simulink model "Test_FourMotor_PID_Ave"  (R2025a)
settings: Solver=ode4  StartTime=0.0  StopTime=2  FixedStep=60e-6  RelTol=1e-3
values from neighbouring files (symbols this model uses):
  Ts = 2e-6    (= 2e-06)    [param.m]
  ts_vec = 60e-6    (= 6e-05)    [param.m]
undefined symbols (not defined in the file or in its folder): DiscIntNeverNeededParam, gcbh, HEV_Param, Limit, magnitude, motorctrl, RPM, sps_rtmsupport
libraries: fl_lib x39, spsCurrentMeasurementLib x26, spsIdealSwitchLib x24, nesl_utility x22, spsVoltageMeasurementLib x21, simulink_extras x13, spsControlledCurrentSourceLib x12, spsControlledVoltageSourceLib x9, slpidlib x7, simulink x6, Uav_Electrical_lib x5, spsSeriesRLCBranchLib x4
(part 3 of 5)

== system Test_FourMotor_PID_Ave/Detailed/Synchronous Motor & Drive1/Torque limitation ==
  N rad/s : Inport
  Torque : Inport  Port=2
  Abs1 : Abs
  Gain : Gain  Gain=-1
  Saturation Dynamic : simulink/Discontinuities/Saturation Dynamic  OutMin=[]  OutMax=[]  OutDataTypeStr=Inherit: Same as second input  OutDataType=sfix(16)  OutScaling=2^-10  DoSatur=off
  Torque vs speed profile : Lookup  InputValues=HEV_Param.Motor.TorqSpdLUT.SpeedRPM*pi/30  Table=HEV_Param.Motor.TorqSpdLUT.TorqueNm  LookUpMeth=Interpolation-Use End Values  SaturateOnIntegerOverflow=off
  torque : Outport  VectorParamsAs1DForOutWhenUnconnected=off
  wires:
  Gain/1 -> Saturation Dynamic/3
  Torque/1 -> Saturation Dynamic/2
  Saturation Dynamic/1 -> torque/1
  Torque vs speed profile/1 -> Gain/1, Saturation Dynamic/1
  Abs1/1 -> Torque vs speed profile/1
  N rad/s/1 -> Abs1/1

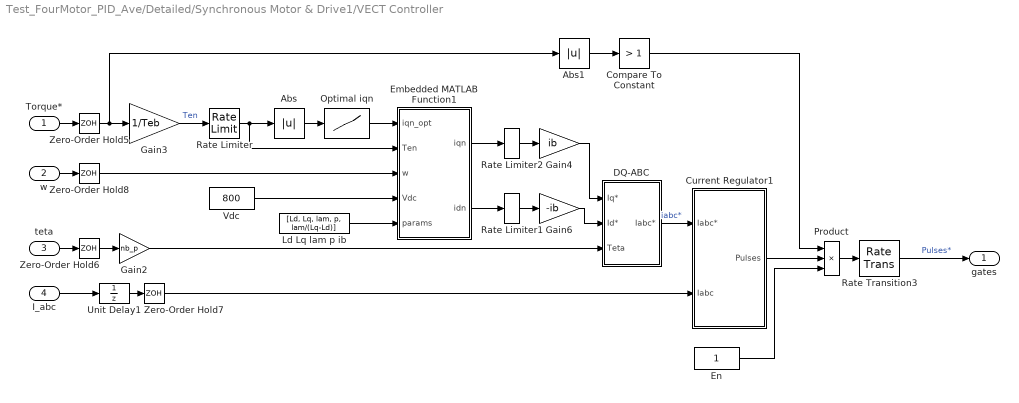
== system Test_FourMotor_PID_Ave/Detailed/Synchronous Motor & Drive1/VECT Controller ==
  Torque* : Inport
  w : Inport  Port=2
  teta : Inport  Port=3
  I_abc : Inport  Port=4
  Abs : Abs  SaturateOnIntegerOverflow=off
  Abs1 : Abs  SaturateOnIntegerOverflow=off
  Compare To Constant : simulink/Logic and Bit Operations/Compare To Constant  relop=>  const=1  OutDataTypeStr=uint8
  Current Regulator1 : Subsystem
  DQ-ABC : Subsystem
  Embedded MATLAB Function1 : MATLAB Function  TreatAsAtomicUnit=on  SystemSampleTime=Ts_vect
  En : Constant
  Gain2 : Gain  Gain=nb_p  SaturateOnIntegerOverflow=on  OutDataTypeStr=Inherit: Same as input  ParamDataTypeStr=Inherit: Same as input
  Gain3 : Gain  Gain=1/Teb  SaturateOnIntegerOverflow=on  OutDataTypeStr=Inherit: Same as input  ParamDataTypeStr=Inherit: Same as input
  Gain4 : Gain  Gain=ib  SaturateOnIntegerOverflow=on  OutDataTypeStr=Inherit: Same as input  ParamDataTypeStr=Inherit: Same as input
  Gain6 : Gain  Gain=-ib  SaturateOnIntegerOverflow=on  OutDataTypeStr=Inherit: Same as input  ParamDataTypeStr=Inherit: Same as input
  Ld Lq lam p ib : Constant  Value=[Ld, Lq, lam, p, lam/(Lq-Ld)]
  Optimal iqn : Lookup  InputValues=ten  Table=iqn  SaturateOnIntegerOverflow=off
  Product : Product  Inputs=3  RndMeth=Zero
  Rate Limiter : RateLimiter  RisingSlewLimit=10  FallingSlewLimit=-10  LinearizeAsGain=off
  Rate Limiter1 : RateLimiter  RisingSlewLimit=100  FallingSlewLimit=-100  SampleTimeMode=inherited
  Rate Limiter2 : RateLimiter  RisingSlewLimit=100  FallingSlewLimit=-100  SampleTimeMode=inherited
  Rate Transition3 : RateTransition
  Unit Delay1 : UnitDelay  SampleTime=-1  HasFrameUpgradeWarning=on
  Vdc : Constant  Value=800
  Zero-Order Hold{5..8} (4 alike) : ZeroOrderHold  SampleTime=Ts_vect
  gates : Outport  VectorParamsAs1DForOutWhenUnconnected=off
  wires:
  Abs1/1 -> Compare To Constant/1
  Compare To Constant/1 -> Product/1
  En/1 -> Product/3
  Current Regulator1/1(Pulses) -> Product/2
  Unit Delay1/1 -> Zero-Order Hold7/1
  Zero-Order Hold7/1 -> Current Regulator1/2(Iabc)
  teta/1 -> Zero-Order Hold6/1
  Zero-Order Hold6/1 -> Gain2/1
  Gain2/1 -> DQ-ABC/3(Teta)
  DQ-ABC/1(Iabc*) -> Current Regulator1/1(Iabc*)  "iabc*"
  I_abc/1 -> Unit Delay1/1
  Torque*/1 -> Zero-Order Hold5/1
  Gain4/1 -> DQ-ABC/1("Iq* ")
  Gain6/1 -> DQ-ABC/2("Id* ")
  Zero-Order Hold5/1 -> Abs1/1, Gain3/1
  w/1 -> Zero-Order Hold8/1
  Embedded MATLAB Function1/2(idn) -> Rate Limiter1/1
  Gain3/1 -> Rate Limiter/1  "Ten"
  Zero-Order Hold8/1 -> Embedded MATLAB Function1/3(w)
  Ld Lq lam p ib/1 -> Embedded MATLAB Function1/5(params)
  Embedded MATLAB Function1/1(iqn) -> Rate Limiter2/1
  Optimal iqn/1 -> Embedded MATLAB Function1/1(iqn_opt)
  Abs/1 -> Optimal iqn/1
  Vdc/1 -> Embedded MATLAB Function1/4(Vdc)
  Rate Transition3/1 -> gates/1  "Pulses*"
  Product/1 -> Rate Transition3/1
  Rate Limiter2/1 -> Gain4/1
  Rate Limiter1/1 -> Gain6/1
  Rate Limiter/1 -> Abs/1, Embedded MATLAB Function1/2(Ten)

== system Test_FourMotor_PID_Ave/Detailed/Synchronous Motor & Drive2/GF ==
  In1 : Inport
  Out1 : Outport  VectorParamsAs1DForOutWhenUnconnected=off
  tag scope: Mot_TReq_SYS_2=global
  wires:
  In1/1 -> Out1/1, [Mot_TReq_SYS_2]

== system Test_FourMotor_PID_Ave/Detailed/Synchronous Motor & Drive2/Measures ==
  Current Measurement : spsCurrentMeasurementLib/Current Measurement  Tag=PoWeRsYsTeMmEaSuReMeNt  PhasorSimulation=off  OutputType=Magnitude  PSBequivalent=0
      settings: AttributesFormatString=\n
  Current Measurement1 : spsCurrentMeasurementLib/Current Measurement  Tag=PoWeRsYsTeMmEaSuReMeNt  PhasorSimulation=off  OutputType=Magnitude  PSBequivalent=0
      settings: AttributesFormatString=\n
  Current Measurement2 : spsCurrentMeasurementLib/Current Measurement  Tag=PoWeRsYsTeMmEaSuReMeNt  PhasorSimulation=off  OutputType=Magnitude  PSBequivalent=0
      settings: AttributesFormatString=\n
  Mux1 : Mux  Inputs=3
  Ta : PMIOPort  Side=Left
  Tb : PMIOPort  Port=2  Side=Left
  Tc : PMIOPort  Port=3  Side=Left
  Mta : PMIOPort  Port=4  Side=Right
  Mtb : PMIOPort  Port=5  Side=Right
  Mtc : PMIOPort  Port=6  Side=Right
  I_abc : Outport  VectorParamsAs1DForOutWhenUnconnected=off
  wires:
  Current Measurement1/1 -> Mux1/2
  Current Measurement/1 -> Mux1/1
  Current Measurement2/1 -> Mux1/3
  Mux1/1 -> I_abc/1
  connections:
  Current Measurement1/RConn1 -- Mtb/RConn1
  Tb/RConn1 -- Current Measurement1/LConn1
  Current Measurement/RConn1 -- Mta/RConn1
  Ta/RConn1 -- Current Measurement/LConn1
  Tc/RConn1 -- Current Measurement2/LConn1
  Current Measurement2/RConn1 -- Mtc/RConn1

== system Test_FourMotor_PID_Ave/Detailed/Synchronous Motor & Drive2/Subsystem ==
  In : Inport
  "+ -> -1" : Gain  Gain=30/pi
  Bus Selector : BusSelector  OutputSignals=Stator current is_a (A),Rotor speed wm (rad/s),Electromagnetic torque Te (N*m)
  Mux1 : Mux  Inputs=2
  Mux2 : Mux  Inputs=3
  Out : Outport  VectorParamsAs1DForOutWhenUnconnected=off
  tag scope: MotorDrive_2=global
  wires:
  In/1 -> Bus Selector/1, Out/1
  "+ -> -1"/1 -> Mux2/2
  [Mot_TReq_SYS_2] -> Mux1/2
  Bus Selector/2 -> "+ -> -1"/1  "<Rotor speed wm (rad/s)>"
  Bus Selector/3 -> Mux1/1  "<Electromagnetic torque Te (N*m)>"
  Mux1/1 -> Mux2/3
  Bus Selector/1 -> Mux2/1  "<Stator current is_a (A)>"
  Mux2/1 -> [MotorDrive_2]

== system Test_FourMotor_PID_Ave/Detailed/Synchronous Motor & Drive2/Subsystem1 ==
  Sig : Inport
  Bus Selector : BusSelector  OutputSignals=Electromagnetic torque Te (N*m)
  Ideal Rotational Motion Sensor : fl_lib/Mechanical/Mechanical Sensors/Ideal Rotational Motion Sensor  reference=foundation.enum.MeasurementReference.difference  acceleration_port=false  velocity_port=true  position_port=true  wrap_angle=simscape.enum.onoff.off  offset=0 rad
  Ideal Torque Source : fl_lib/Mechanical/Mechanical Sources/Ideal Torque Source
  Mechanical Rotational Reference : fl_lib/Mechanical/Rotational Elements/Mechanical Rotational Reference
  Mechanical Rotational Reference1 : fl_lib/Mechanical/Rotational Elements/Mechanical Rotational Reference
  PS-Simulink Converter : nesl_utility/PS-Simulink Converter  PhysicalDomain=network_engine_domain  SubClassName=ps_output  LeftPortType=input  RightPortType=output  PseudoPeriodic=off  Frequencies=[]  VectorFormat=1-D array  Unit=rad/s  AffineConversion=off
  Scope : Scope
      settings: ActiveDisplayYMinimum=-14.945816065975556  ActiveDisplayYMaximum=38.271093163037733  DataLoggingVariableName=ScopeData6
  Simulink-PS Converter : nesl_utility/Simulink-PS Converter  PhysicalDomain=network_engine_domain  SubClassName=ps_input  LeftPortType=input  RightPortType=output  PseudoPeriodic=off  Frequencies=[]  NoiseDistribution=none  NoiseParameters=[]  Unit=1  AffineConversion=off  FilteringAndDerivatives=zero  SimscapeFilterOrder=1  InputFilterTimeConstant=0.005  UdotUserProvided=0
  Sh : PMIOPort  Side=Right
  Spd : Outport  VectorParamsAs1DForOutWhenUnconnected=off
  wires:
  PS-Simulink Converter/1 -> Spd/1
  Sig/1 -> Bus Selector/1
  Bus Selector/1 -> Scope/1, Simulink-PS Converter/1  "<Electromagnetic torque Te (N*m)>"
  connections:
  Simulink-PS Converter/RConn1 -- Ideal Torque Source/RConn1
  PS-Simulink Converter/LConn1 -- Ideal Rotational Motion Sensor/RConn2
  Ideal Rotational Motion Sensor/LConn1 -- Sh/RConn1 -- Ideal Torque Source/LConn1
  Mechanical Rotational Reference1/LConn1 -- Ideal Torque Source/RConn2
  Mechanical Rotational Reference/LConn1 -- Ideal Rotational Motion Sensor/RConn1

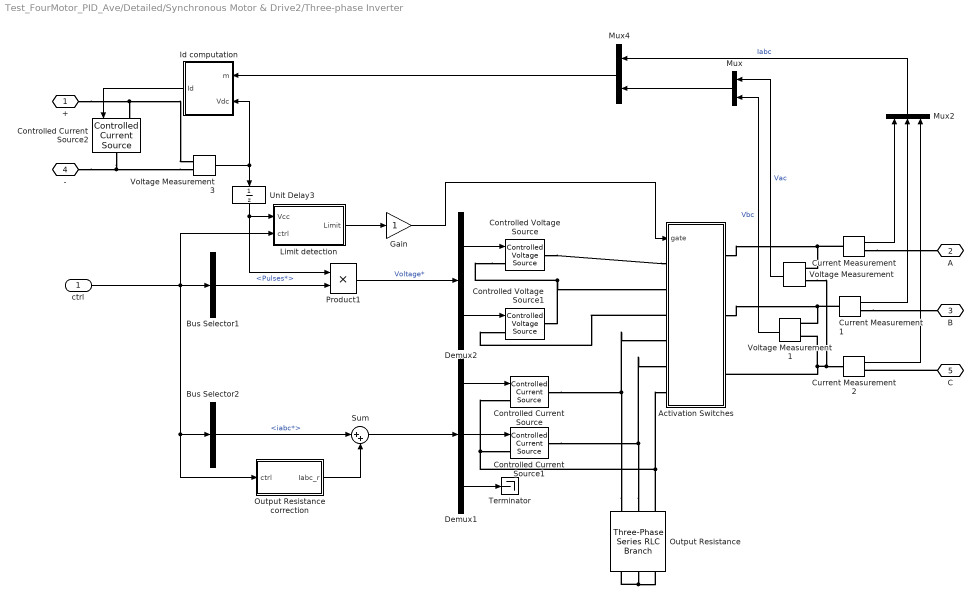
== system Test_FourMotor_PID_Ave/Detailed/Synchronous Motor & Drive2/Three-phase Inverter ==
  ctrl : Inport
  Activation Switches : Subsystem
  Bus Selector1 : BusSelector  OutputSignals=Signals*.Pulses*
  Bus Selector2 : BusSelector  OutputSignals=Signals*.iabc*
  Controlled Current Source : spsControlledCurrentSourceLib/Controlled Current Source  Initialize=on  Source_Type=AC  Amplitude=0  Phase=0  Frequency=0  Measurements=None
  Controlled Current Source1 : spsControlledCurrentSourceLib/Controlled Current Source  Initialize=on  Source_Type=AC  Amplitude=0  Phase=0  Frequency=0  Measurements=None
  Controlled Current Source2 : spsControlledCurrentSourceLib/Controlled Current Source  Initialize=on  Source_Type=AC  Amplitude=0  Phase=0  Frequency=0  Measurements=None
  Controlled Voltage Source : spsControlledVoltageSourceLib/Controlled Voltage Source  Initialize=on  Source_Type=AC  Amplitude=0  Phase=0  Frequency=0  Measurements=None
  Controlled Voltage Source1 : spsControlledVoltageSourceLib/Controlled Voltage Source  Initialize=on  Source_Type=AC  Amplitude=0  Phase=0  Frequency=0  Measurements=None
  Current Measurement : spsCurrentMeasurementLib/Current Measurement  PhasorSimulation=off  OutputType=Complex  PSBequivalent=0
  Current Measurement1 : spsCurrentMeasurementLib/Current Measurement  PhasorSimulation=off  OutputType=Complex  PSBequivalent=0
  Current Measurement2 : spsCurrentMeasurementLib/Current Measurement  PhasorSimulation=off  OutputType=Complex  PSBequivalent=0
  Demux1 : Demux  Outputs=3
      settings: DisplayOption=none
  Demux2 : Demux  Outputs=2
      settings: DisplayOption=none
  Gain : Gain
  Id computation : Subsystem
  Limit detection : Subsystem
  Mux : Mux  Inputs=2
  Mux2 : Mux  Inputs=3
  Mux4 : Mux  Inputs=2
  Output Resistance : spsThreePhaseSeriesRLCBranchLib/Three-Phase Series RLC Branch  LConnTagsString=A|B|C  RConnTagsString=A|B|C  BranchType=R  Resistance=100*Resistance  Inductance=1e-3  Capacitance=1e-6  Measurements=Branch voltages and currents
  Output Resistance correction : Subsystem
  Product1 : Product  RndMeth=Zero
  Sum : Sum  Inputs=|++
  Terminator : Terminator
  Unit Delay3 : UnitDelay  SampleTime=Ts  HasFrameUpgradeWarning=on
  Voltage Measurement : spsVoltageMeasurementLib/Voltage Measurement  PhasorSimulation=off  OutputType=Complex  PSBequivalent=0
  Voltage Measurement1 : spsVoltageMeasurementLib/Voltage Measurement  PhasorSimulation=off  OutputType=Complex  PSBequivalent=0
  Voltage Measurement3 : spsVoltageMeasurementLib/Voltage Measurement  PhasorSimulation=off  OutputType=Complex  PSBequivalent=0
  + : PMIOPort  Side=Right
  A : PMIOPort  Port=2  Side=Left
  B : PMIOPort  Port=3  Side=Left
  - : PMIOPort  Port=4  Side=Right
  C : PMIOPort  Port=5  Side=Left
  wires:
  Current Measurement/1 -> Mux2/1
  Current Measurement1/1 -> Mux2/2
  Voltage Measurement/1 -> Mux/1  "Vac"
  Voltage Measurement1/1 -> Mux/2  "Vbc"
  Mux/1 -> Mux4/2
  Current Measurement2/1 -> Mux2/3
  Mux4/1 -> Id computation/1(m)
  Mux2/1 -> Mux4/1  "Iabc"
  Voltage Measurement3/1 -> Unit Delay3/1, Id computation/2(Vdc)
  Bus Selector1/1 -> Product1/2  "<Pulses*>"
  Demux1/1 -> Controlled Current Source/1
  Demux1/2 -> Controlled Current Source1/1
  Demux1/3 -> Terminator/1
  Demux2/2 -> Controlled Voltage Source1/1
  Demux2/1 -> Controlled Voltage Source/1
  Bus Selector2/1 -> Sum/1  "<iabc*>"
  Limit detection/1(Limit) -> Gain/1
  Sum/1 -> Demux1/1
  Unit Delay3/1 -> Product1/1, Limit detection/1(Vcc)
  ctrl/1 -> Bus Selector1/1, Limit detection/2(ctrl), Bus Selector2/1, Output Resistance correction/1(ctrl)
  Product1/1 -> Demux2/1  "Voltage*"
  Gain/1 -> Activation Switches/1(gate)
  Id computation/1(Id) -> Controlled Current Source2/1
  Output Resistance correction/1("Iabc_r ") -> Sum/2
  connections:
  Voltage Measurement3/LConn1 -- Controlled Current Source2/LConn1 -- +/RConn1
  Voltage Measurement3/LConn2 -- Controlled Current Source2/RConn1 -- -/RConn1
  Activation Switches/LConn6 -- Controlled Current Source/LConn1 -- Controlled Current Source1/LConn1 -- Output Resistance/LConn3
  Output Resistance/RConn1 -- Output Resistance/RConn3 -- Output Resistance/RConn2
  Voltage Measurement/LConn1 -- Activation Switches/RConn1 -- Current Measurement/LConn1
  Output Resistance/LConn1 -- Activation Switches/LConn4 -- Controlled Current Source/RConn1
  Output Resistance/LConn2 -- Activation Switches/LConn5 -- Controlled Current Source1/RConn1
  Voltage Measurement/LConn2 -- Activation Switches/RConn3 -- Voltage Measurement1/LConn2 -- Current Measurement2/LConn1
  Controlled Voltage Source/LConn1 -- Activation Switches/LConn2 -- Controlled Voltage Source1/RConn1
  Voltage Measurement1/LConn1 -- Activation Switches/RConn2 -- Current Measurement1/LConn1
  Current Measurement/RConn1 -- A/RConn1
  Current Measurement1/RConn1 -- B/RConn1
  C/RConn1 -- Current Measurement2/RConn1
  Controlled Voltage Source/RConn1 -- Activation Switches/LConn1
  Activation Switches/LConn3 -- Controlled Voltage Source1/LConn1

== system Test_FourMotor_PID_Ave/Detailed/Synchronous Motor & Drive2/Torque limitation ==
  N rad/s : Inport
  Torque : Inport  Port=2
  Abs1 : Abs
  Gain : Gain  Gain=-1
  Saturation Dynamic : simulink/Discontinuities/Saturation Dynamic  OutMin=[]  OutMax=[]  OutDataTypeStr=Inherit: Same as second input  OutDataType=sfix(16)  OutScaling=2^-10  DoSatur=off
  Torque vs speed profile : Lookup  InputValues=HEV_Param.Motor.TorqSpdLUT.SpeedRPM*pi/30  Table=HEV_Param.Motor.TorqSpdLUT.TorqueNm  LookUpMeth=Interpolation-Use End Values  SaturateOnIntegerOverflow=off
  torque : Outport  VectorParamsAs1DForOutWhenUnconnected=off
  wires:
  Gain/1 -> Saturation Dynamic/3
  Torque/1 -> Saturation Dynamic/2
  Saturation Dynamic/1 -> torque/1
  Torque vs speed profile/1 -> Gain/1, Saturation Dynamic/1
  Abs1/1 -> Torque vs speed profile/1
  N rad/s/1 -> Abs1/1

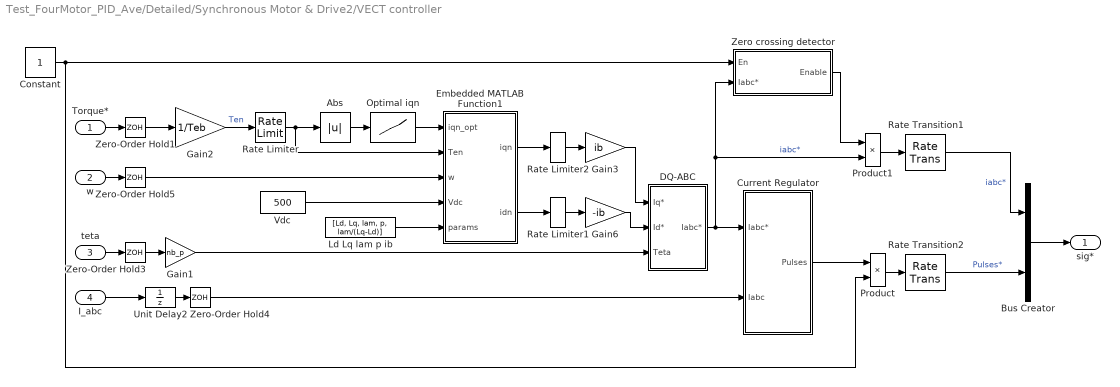
== system Test_FourMotor_PID_Ave/Detailed/Synchronous Motor & Drive2/VECT controller ==
  Torque* : Inport
  w : Inport  Port=2
  teta : Inport  Port=3
  I_abc : Inport  Port=4
  Abs : Abs  SaturateOnIntegerOverflow=off
  Bus Creator : BusCreator  Inputs=2
  Constant : Constant
  Current Regulator : Subsystem
  DQ-ABC : Subsystem
  Embedded MATLAB Function1 : MATLAB Function  TreatAsAtomicUnit=on  SystemSampleTime=Ts_vect
  Gain1 : Gain  Gain=nb_p  SaturateOnIntegerOverflow=on  OutDataTypeStr=Inherit: Same as input  ParamDataTypeStr=Inherit: Same as input
  Gain2 : Gain  Gain=1/Teb  SaturateOnIntegerOverflow=on  OutDataTypeStr=Inherit: Same as input  ParamDataTypeStr=Inherit: Same as input
  Gain3 : Gain  Gain=ib  SaturateOnIntegerOverflow=on  OutDataTypeStr=Inherit: Same as input  ParamDataTypeStr=Inherit: Same as input
  Gain6 : Gain  Gain=-ib  SaturateOnIntegerOverflow=on  OutDataTypeStr=Inherit: Same as input  ParamDataTypeStr=Inherit: Same as input
  Ld Lq lam p ib : Constant  Value=[Ld, Lq, lam, p, lam/(Lq-Ld)]
  Optimal iqn : Lookup  InputValues=ten  Table=iqn  SaturateOnIntegerOverflow=off
  Product : Product  RndMeth=Zero
  Product1 : Product  RndMeth=Zero
  Rate Limiter : RateLimiter  RisingSlewLimit=10  FallingSlewLimit=-10  LinearizeAsGain=off
  Rate Limiter1 : RateLimiter  RisingSlewLimit=100  FallingSlewLimit=-100  SampleTimeMode=inherited
  Rate Limiter2 : RateLimiter  RisingSlewLimit=100  FallingSlewLimit=-100  SampleTimeMode=inherited
  Rate Transition1 : RateTransition
  Rate Transition2 : RateTransition
  Unit Delay2 : UnitDelay  SampleTime=-1  HasFrameUpgradeWarning=on
  Vdc : Constant  Value=500
  Zero crossing detector : Subsystem
  Zero-Order Hold{1,3..5} (4 alike) : ZeroOrderHold  SampleTime=Ts_vect
  sig* : Outport  VectorParamsAs1DForOutWhenUnconnected=off
  wires:
  Unit Delay2/1 -> Zero-Order Hold4/1
  Zero-Order Hold4/1 -> Current Regulator/2(Iabc)
  teta/1 -> Zero-Order Hold3/1
  Zero-Order Hold3/1 -> Gain1/1
  Gain1/1 -> DQ-ABC/3(Teta)
  DQ-ABC/1(Iabc*) -> Current Regulator/1(Iabc*), Zero crossing detector/2(Iabc*), Product1/2  "iabc*"
  I_abc/1 -> Unit Delay2/1
  Torque*/1 -> Zero-Order Hold1/1
  Gain3/1 -> DQ-ABC/1("Iq* ")
  Gain6/1 -> DQ-ABC/2("Id* ")
  Zero-Order Hold1/1 -> Gain2/1
  w/1 -> Zero-Order Hold5/1
  Embedded MATLAB Function1/2(idn) -> Rate Limiter1/1
  Gain2/1 -> Rate Limiter/1  "Ten"
  Zero-Order Hold5/1 -> Embedded MATLAB Function1/3(w)
  Ld Lq lam p ib/1 -> Embedded MATLAB Function1/5(params)
  Embedded MATLAB Function1/1(iqn) -> Rate Limiter2/1
  Optimal iqn/1 -> Embedded MATLAB Function1/1(iqn_opt)
  Abs/1 -> Optimal iqn/1
  Vdc/1 -> Embedded MATLAB Function1/4(Vdc)
  Bus Creator/1 -> sig*/1
  Rate Transition2/1 -> Bus Creator/2  "Pulses*"
  Rate Transition1/1 -> Bus Creator/1  "iabc*"
  Current Regulator/1(Pulses) -> Product/1
  Product/1 -> Rate Transition2/1
  Product1/1 -> Rate Transition1/1
  Zero crossing detector/1(Enable) -> Product1/1
  Constant/1 -> Zero crossing detector/1(En), Product/2
  Rate Limiter2/1 -> Gain3/1
  Rate Limiter1/1 -> Gain6/1
  Rate Limiter/1 -> Abs/1, Embedded MATLAB Function1/2(Ten)

== system Test_FourMotor_PID_Ave/Detailed/Synchronous Motor & Drive3/GF ==
  In1 : Inport
  Out1 : Outport  VectorParamsAs1DForOutWhenUnconnected=off
  tag scope: Mot_TReq_SYS_3=global
  wires:
  In1/1 -> Out1/1, [Mot_TReq_SYS_3]

== system Test_FourMotor_PID_Ave/Detailed/Synchronous Motor & Drive3/Measures ==
  Current Measurement : spsCurrentMeasurementLib/Current Measurement  Tag=PoWeRsYsTeMmEaSuReMeNt  PhasorSimulation=off  OutputType=Magnitude  PSBequivalent=0
      settings: AttributesFormatString=\n
  Current Measurement1 : spsCurrentMeasurementLib/Current Measurement  Tag=PoWeRsYsTeMmEaSuReMeNt  PhasorSimulation=off  OutputType=Magnitude  PSBequivalent=0
      settings: AttributesFormatString=\n
  Current Measurement2 : spsCurrentMeasurementLib/Current Measurement  Tag=PoWeRsYsTeMmEaSuReMeNt  PhasorSimulation=off  OutputType=Magnitude  PSBequivalent=0
      settings: AttributesFormatString=\n
  Mux1 : Mux  Inputs=3
  Ta : PMIOPort  Side=Left
  Tb : PMIOPort  Port=2  Side=Left
  Tc : PMIOPort  Port=3  Side=Left
  Mta : PMIOPort  Port=4  Side=Right
  Mtb : PMIOPort  Port=5  Side=Right
  Mtc : PMIOPort  Port=6  Side=Right
  I_abc : Outport  VectorParamsAs1DForOutWhenUnconnected=off
  wires:
  Current Measurement1/1 -> Mux1/2
  Current Measurement/1 -> Mux1/1
  Current Measurement2/1 -> Mux1/3
  Mux1/1 -> I_abc/1
  connections:
  Current Measurement1/RConn1 -- Mtb/RConn1
  Tb/RConn1 -- Current Measurement1/LConn1
  Current Measurement/RConn1 -- Mta/RConn1
  Ta/RConn1 -- Current Measurement/LConn1
  Tc/RConn1 -- Current Measurement2/LConn1
  Current Measurement2/RConn1 -- Mtc/RConn1

== system Test_FourMotor_PID_Ave/Detailed/Synchronous Motor & Drive3/Subsystem ==
  In : Inport
  "+ -> -1" : Gain  Gain=30/pi
  Bus Selector : BusSelector  OutputSignals=Stator current is_a (A),Rotor speed wm (rad/s),Electromagnetic torque Te (N*m)
  Mux1 : Mux  Inputs=2
  Mux2 : Mux  Inputs=3
  Out : Outport  VectorParamsAs1DForOutWhenUnconnected=off
  tag scope: MotorDrive_3=global
  wires:
  In/1 -> Bus Selector/1, Out/1
  "+ -> -1"/1 -> Mux2/2
  [Mot_TReq_SYS_3] -> Mux1/2
  Bus Selector/2 -> "+ -> -1"/1  "<Rotor speed wm (rad/s)>"
  Bus Selector/3 -> Mux1/1  "<Electromagnetic torque Te (N*m)>"
  Mux1/1 -> Mux2/3
  Bus Selector/1 -> Mux2/1  "<Stator current is_a (A)>"
  Mux2/1 -> [MotorDrive_3]

== system Test_FourMotor_PID_Ave/Detailed/Synchronous Motor & Drive3/Subsystem1 ==
  Sig : Inport
  Bus Selector : BusSelector  OutputSignals=Electromagnetic torque Te (N*m)
  Ideal Rotational Motion Sensor : fl_lib/Mechanical/Mechanical Sensors/Ideal Rotational Motion Sensor  reference=foundation.enum.MeasurementReference.difference  acceleration_port=false  velocity_port=true  position_port=true  wrap_angle=simscape.enum.onoff.off  offset=0 rad
  Ideal Torque Source : fl_lib/Mechanical/Mechanical Sources/Ideal Torque Source
  Mechanical Rotational Reference : fl_lib/Mechanical/Rotational Elements/Mechanical Rotational Reference
  Mechanical Rotational Reference1 : fl_lib/Mechanical/Rotational Elements/Mechanical Rotational Reference
  PS-Simulink Converter : nesl_utility/PS-Simulink Converter  PhysicalDomain=network_engine_domain  SubClassName=ps_output  LeftPortType=input  RightPortType=output  PseudoPeriodic=off  Frequencies=[]  VectorFormat=1-D array  Unit=rad/s  AffineConversion=off
  Scope : Scope
      settings: ActiveDisplayYMinimum=-14.945816065975556  ActiveDisplayYMaximum=38.271093163037733  DataLoggingVariableName=ScopeData6
  Simulink-PS Converter : nesl_utility/Simulink-PS Converter  PhysicalDomain=network_engine_domain  SubClassName=ps_input  LeftPortType=input  RightPortType=output  PseudoPeriodic=off  Frequencies=[]  NoiseDistribution=none  NoiseParameters=[]  Unit=1  AffineConversion=off  FilteringAndDerivatives=zero  SimscapeFilterOrder=1  InputFilterTimeConstant=0.005  UdotUserProvided=0
  Sh : PMIOPort  Side=Right
  Spd : Outport  VectorParamsAs1DForOutWhenUnconnected=off
  wires:
  PS-Simulink Converter/1 -> Spd/1
  Sig/1 -> Bus Selector/1
  Bus Selector/1 -> Scope/1, Simulink-PS Converter/1  "<Electromagnetic torque Te (N*m)>"
  connections:
  Simulink-PS Converter/RConn1 -- Ideal Torque Source/RConn1
  PS-Simulink Converter/LConn1 -- Ideal Rotational Motion Sensor/RConn2
  Ideal Rotational Motion Sensor/LConn1 -- Sh/RConn1 -- Ideal Torque Source/LConn1
  Mechanical Rotational Reference1/LConn1 -- Ideal Torque Source/RConn2
  Mechanical Rotational Reference/LConn1 -- Ideal Rotational Motion Sensor/RConn1

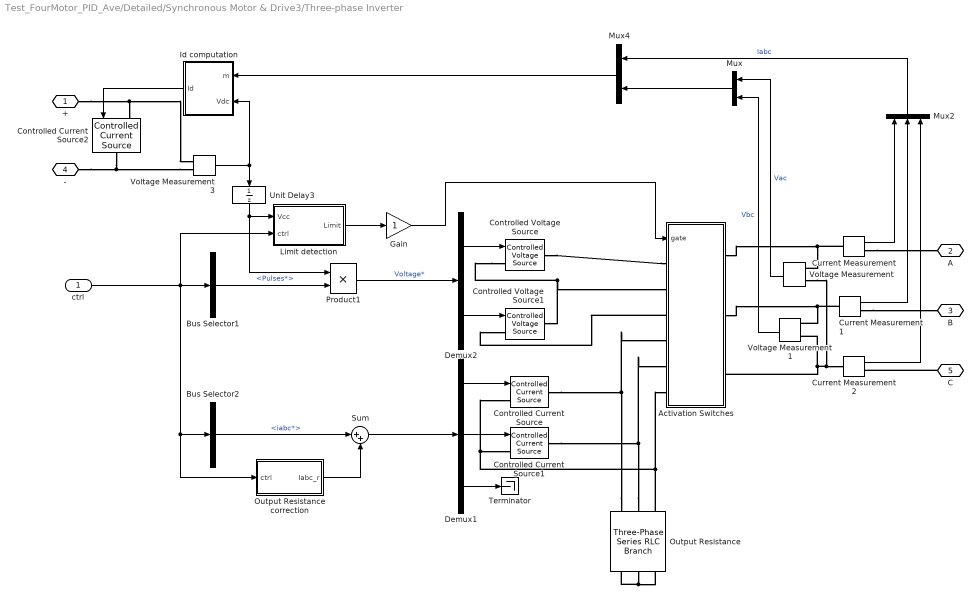
== system Test_FourMotor_PID_Ave/Detailed/Synchronous Motor & Drive3/Three-phase Inverter ==
  ctrl : Inport
  Activation Switches : Subsystem
  Bus Selector1 : BusSelector  OutputSignals=Signals*.Pulses*
  Bus Selector2 : BusSelector  OutputSignals=Signals*.iabc*
  Controlled Current Source : spsControlledCurrentSourceLib/Controlled Current Source  Initialize=on  Source_Type=AC  Amplitude=0  Phase=0  Frequency=0  Measurements=None
  Controlled Current Source1 : spsControlledCurrentSourceLib/Controlled Current Source  Initialize=on  Source_Type=AC  Amplitude=0  Phase=0  Frequency=0  Measurements=None
  Controlled Current Source2 : spsControlledCurrentSourceLib/Controlled Current Source  Initialize=on  Source_Type=AC  Amplitude=0  Phase=0  Frequency=0  Measurements=None
  Controlled Voltage Source : spsControlledVoltageSourceLib/Controlled Voltage Source  Initialize=on  Source_Type=AC  Amplitude=0  Phase=0  Frequency=0  Measurements=None
  Controlled Voltage Source1 : spsControlledVoltageSourceLib/Controlled Voltage Source  Initialize=on  Source_Type=AC  Amplitude=0  Phase=0  Frequency=0  Measurements=None
  Current Measurement : spsCurrentMeasurementLib/Current Measurement  PhasorSimulation=off  OutputType=Complex  PSBequivalent=0
  Current Measurement1 : spsCurrentMeasurementLib/Current Measurement  PhasorSimulation=off  OutputType=Complex  PSBequivalent=0
  Current Measurement2 : spsCurrentMeasurementLib/Current Measurement  PhasorSimulation=off  OutputType=Complex  PSBequivalent=0
  Demux1 : Demux  Outputs=3
      settings: DisplayOption=none
  Demux2 : Demux  Outputs=2
      settings: DisplayOption=none
  Gain : Gain
  Id computation : Subsystem
  Limit detection : Subsystem
  Mux : Mux  Inputs=2
  Mux2 : Mux  Inputs=3
  Mux4 : Mux  Inputs=2
  Output Resistance : spsThreePhaseSeriesRLCBranchLib/Three-Phase Series RLC Branch  LConnTagsString=A|B|C  RConnTagsString=A|B|C  BranchType=R  Resistance=100*Resistance  Inductance=1e-3  Capacitance=1e-6  Measurements=Branch voltages and currents
  Output Resistance correction : Subsystem
  Product1 : Product  RndMeth=Zero
  Sum : Sum  Inputs=|++
  Terminator : Terminator
  Unit Delay3 : UnitDelay  SampleTime=Ts  HasFrameUpgradeWarning=on
  Voltage Measurement : spsVoltageMeasurementLib/Voltage Measurement  PhasorSimulation=off  OutputType=Complex  PSBequivalent=0
  Voltage Measurement1 : spsVoltageMeasurementLib/Voltage Measurement  PhasorSimulation=off  OutputType=Complex  PSBequivalent=0
  Voltage Measurement3 : spsVoltageMeasurementLib/Voltage Measurement  PhasorSimulation=off  OutputType=Complex  PSBequivalent=0
  + : PMIOPort  Side=Right
  A : PMIOPort  Port=2  Side=Left
  B : PMIOPort  Port=3  Side=Left
  - : PMIOPort  Port=4  Side=Right
  C : PMIOPort  Port=5  Side=Left
  wires:
  Current Measurement/1 -> Mux2/1
  Current Measurement1/1 -> Mux2/2
  Voltage Measurement/1 -> Mux/1  "Vac"
  Voltage Measurement1/1 -> Mux/2  "Vbc"
  Mux/1 -> Mux4/2
  Current Measurement2/1 -> Mux2/3
  Mux4/1 -> Id computation/1(m)
  Mux2/1 -> Mux4/1  "Iabc"
  Voltage Measurement3/1 -> Unit Delay3/1, Id computation/2(Vdc)
  Bus Selector1/1 -> Product1/2  "<Pulses*>"
  Demux1/1 -> Controlled Current Source/1
  Demux1/2 -> Controlled Current Source1/1
  Demux1/3 -> Terminator/1
  Demux2/2 -> Controlled Voltage Source1/1
  Demux2/1 -> Controlled Voltage Source/1
  Bus Selector2/1 -> Sum/1  "<iabc*>"
  Limit detection/1(Limit) -> Gain/1
  Sum/1 -> Demux1/1
  Unit Delay3/1 -> Product1/1, Limit detection/1(Vcc)
  ctrl/1 -> Bus Selector1/1, Limit detection/2(ctrl), Bus Selector2/1, Output Resistance correction/1(ctrl)
  Product1/1 -> Demux2/1  "Voltage*"
  Gain/1 -> Activation Switches/1(gate)
  Id computation/1(Id) -> Controlled Current Source2/1
  Output Resistance correction/1("Iabc_r ") -> Sum/2
  connections:
  Voltage Measurement3/LConn1 -- Controlled Current Source2/LConn1 -- +/RConn1
  Voltage Measurement3/LConn2 -- Controlled Current Source2/RConn1 -- -/RConn1
  Activation Switches/LConn6 -- Controlled Current Source/LConn1 -- Controlled Current Source1/LConn1 -- Output Resistance/LConn3
  Output Resistance/RConn1 -- Output Resistance/RConn3 -- Output Resistance/RConn2
  Voltage Measurement/LConn1 -- Activation Switches/RConn1 -- Current Measurement/LConn1
  Output Resistance/LConn1 -- Activation Switches/LConn4 -- Controlled Current Source/RConn1
  Output Resistance/LConn2 -- Activation Switches/LConn5 -- Controlled Current Source1/RConn1
  Voltage Measurement/LConn2 -- Activation Switches/RConn3 -- Voltage Measurement1/LConn2 -- Current Measurement2/LConn1
  Controlled Voltage Source/LConn1 -- Activation Switches/LConn2 -- Controlled Voltage Source1/RConn1
  Voltage Measurement1/LConn1 -- Activation Switches/RConn2 -- Current Measurement1/LConn1
  Current Measurement/RConn1 -- A/RConn1
  Current Measurement1/RConn1 -- B/RConn1
  C/RConn1 -- Current Measurement2/RConn1
  Controlled Voltage Source/RConn1 -- Activation Switches/LConn1
  Activation Switches/LConn3 -- Controlled Voltage Source1/LConn1

== system Test_FourMotor_PID_Ave/Detailed/Synchronous Motor & Drive3/Torque limitation ==
  N rad/s : Inport
  Torque : Inport  Port=2
  Abs1 : Abs
  Gain : Gain  Gain=-1
  Saturation Dynamic : simulink/Discontinuities/Saturation Dynamic  OutMin=[]  OutMax=[]  OutDataTypeStr=Inherit: Same as second input  OutDataType=sfix(16)  OutScaling=2^-10  DoSatur=off
  Torque vs speed profile : Lookup  InputValues=HEV_Param.Motor.TorqSpdLUT.SpeedRPM*pi/30  Table=HEV_Param.Motor.TorqSpdLUT.TorqueNm  LookUpMeth=Interpolation-Use End Values  SaturateOnIntegerOverflow=off
  torque : Outport  VectorParamsAs1DForOutWhenUnconnected=off
  wires:
  Gain/1 -> Saturation Dynamic/3
  Torque/1 -> Saturation Dynamic/2
  Saturation Dynamic/1 -> torque/1
  Torque vs speed profile/1 -> Gain/1, Saturation Dynamic/1
  Abs1/1 -> Torque vs speed profile/1
  N rad/s/1 -> Abs1/1

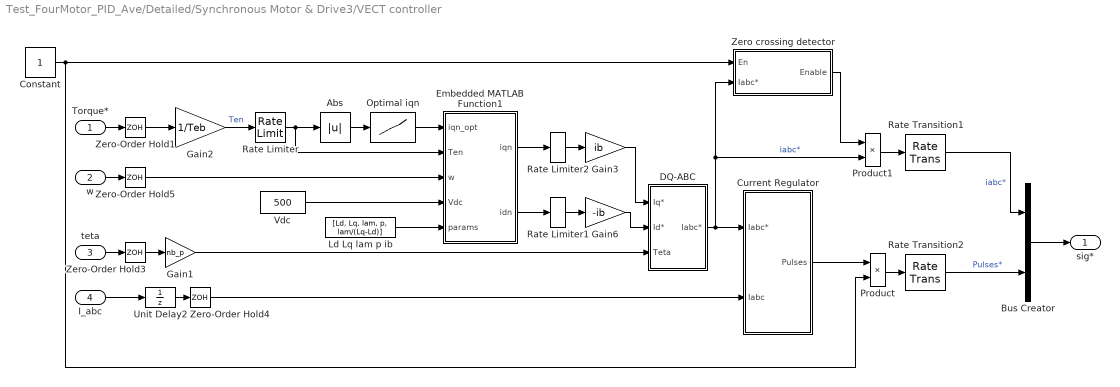
== system Test_FourMotor_PID_Ave/Detailed/Synchronous Motor & Drive3/VECT controller ==
  Torque* : Inport
  w : Inport  Port=2
  teta : Inport  Port=3
  I_abc : Inport  Port=4
  Abs : Abs  SaturateOnIntegerOverflow=off
  Bus Creator : BusCreator  Inputs=2
  Constant : Constant
  Current Regulator : Subsystem
  DQ-ABC : Subsystem
  Embedded MATLAB Function1 : MATLAB Function  TreatAsAtomicUnit=on  SystemSampleTime=Ts_vect
  Gain1 : Gain  Gain=nb_p  SaturateOnIntegerOverflow=on  OutDataTypeStr=Inherit: Same as input  ParamDataTypeStr=Inherit: Same as input
  Gain2 : Gain  Gain=1/Teb  SaturateOnIntegerOverflow=on  OutDataTypeStr=Inherit: Same as input  ParamDataTypeStr=Inherit: Same as input
  Gain3 : Gain  Gain=ib  SaturateOnIntegerOverflow=on  OutDataTypeStr=Inherit: Same as input  ParamDataTypeStr=Inherit: Same as input
  Gain6 : Gain  Gain=-ib  SaturateOnIntegerOverflow=on  OutDataTypeStr=Inherit: Same as input  ParamDataTypeStr=Inherit: Same as input
  Ld Lq lam p ib : Constant  Value=[Ld, Lq, lam, p, lam/(Lq-Ld)]
  Optimal iqn : Lookup  InputValues=ten  Table=iqn  SaturateOnIntegerOverflow=off
  Product : Product  RndMeth=Zero
  Product1 : Product  RndMeth=Zero
  Rate Limiter : RateLimiter  RisingSlewLimit=10  FallingSlewLimit=-10  LinearizeAsGain=off
  Rate Limiter1 : RateLimiter  RisingSlewLimit=100  FallingSlewLimit=-100  SampleTimeMode=inherited
  Rate Limiter2 : RateLimiter  RisingSlewLimit=100  FallingSlewLimit=-100  SampleTimeMode=inherited
  Rate Transition1 : RateTransition
  Rate Transition2 : RateTransition
  Unit Delay2 : UnitDelay  SampleTime=-1  HasFrameUpgradeWarning=on
  Vdc : Constant  Value=500
  Zero crossing detector : Subsystem
  Zero-Order Hold{1,3..5} (4 alike) : ZeroOrderHold  SampleTime=Ts_vect
  sig* : Outport  VectorParamsAs1DForOutWhenUnconnected=off
  wires:
  Unit Delay2/1 -> Zero-Order Hold4/1
  Zero-Order Hold4/1 -> Current Regulator/2(Iabc)
  teta/1 -> Zero-Order Hold3/1
  Zero-Order Hold3/1 -> Gain1/1
  Gain1/1 -> DQ-ABC/3(Teta)
  DQ-ABC/1(Iabc*) -> Current Regulator/1(Iabc*), Zero crossing detector/2(Iabc*), Product1/2  "iabc*"
  I_abc/1 -> Unit Delay2/1
  Torque*/1 -> Zero-Order Hold1/1
  Gain3/1 -> DQ-ABC/1("Iq* ")
  Gain6/1 -> DQ-ABC/2("Id* ")
  Zero-Order Hold1/1 -> Gain2/1
  w/1 -> Zero-Order Hold5/1
  Embedded MATLAB Function1/2(idn) -> Rate Limiter1/1
  Gain2/1 -> Rate Limiter/1  "Ten"
  Zero-Order Hold5/1 -> Embedded MATLAB Function1/3(w)
  Ld Lq lam p ib/1 -> Embedded MATLAB Function1/5(params)
  Embedded MATLAB Function1/1(iqn) -> Rate Limiter2/1
  Optimal iqn/1 -> Embedded MATLAB Function1/1(iqn_opt)
  Abs/1 -> Optimal iqn/1
  Vdc/1 -> Embedded MATLAB Function1/4(Vdc)
  Bus Creator/1 -> sig*/1
  Rate Transition2/1 -> Bus Creator/2  "Pulses*"
  Rate Transition1/1 -> Bus Creator/1  "iabc*"
  Current Regulator/1(Pulses) -> Product/1
  Product/1 -> Rate Transition2/1
  Product1/1 -> Rate Transition1/1
  Zero crossing detector/1(Enable) -> Product1/1
  Constant/1 -> Zero crossing detector/1(En), Product/2
  Rate Limiter2/1 -> Gain3/1
  Rate Limiter1/1 -> Gain6/1
  Rate Limiter/1 -> Abs/1, Embedded MATLAB Function1/2(Ten)

== system Test_FourMotor_PID_Ave/Detailed/Synchronous Motor & Drive4/GF ==
  In1 : Inport
  Out1 : Outport  VectorParamsAs1DForOutWhenUnconnected=off
  tag scope: Mot_TReq_SYS_4=global
  wires:
  In1/1 -> Out1/1, [Mot_TReq_SYS_4]

== system Test_FourMotor_PID_Ave/Detailed/Synchronous Motor & Drive4/Measures ==
  Current Measurement : spsCurrentMeasurementLib/Current Measurement  Tag=PoWeRsYsTeMmEaSuReMeNt  PhasorSimulation=off  OutputType=Magnitude  PSBequivalent=0
      settings: AttributesFormatString=\n
  Current Measurement1 : spsCurrentMeasurementLib/Current Measurement  Tag=PoWeRsYsTeMmEaSuReMeNt  PhasorSimulation=off  OutputType=Magnitude  PSBequivalent=0
      settings: AttributesFormatString=\n
  Current Measurement2 : spsCurrentMeasurementLib/Current Measurement  Tag=PoWeRsYsTeMmEaSuReMeNt  PhasorSimulation=off  OutputType=Magnitude  PSBequivalent=0
      settings: AttributesFormatString=\n
  Mux1 : Mux  Inputs=3
  Ta : PMIOPort  Side=Left
  Tb : PMIOPort  Port=2  Side=Left
  Tc : PMIOPort  Port=3  Side=Left
  Mta : PMIOPort  Port=4  Side=Right
  Mtb : PMIOPort  Port=5  Side=Right
  Mtc : PMIOPort  Port=6  Side=Right
  I_abc : Outport  VectorParamsAs1DForOutWhenUnconnected=off
  wires:
  Current Measurement1/1 -> Mux1/2
  Current Measurement/1 -> Mux1/1
  Current Measurement2/1 -> Mux1/3
  Mux1/1 -> I_abc/1
  connections:
  Current Measurement1/RConn1 -- Mtb/RConn1
  Tb/RConn1 -- Current Measurement1/LConn1
  Current Measurement/RConn1 -- Mta/RConn1
  Ta/RConn1 -- Current Measurement/LConn1
  Tc/RConn1 -- Current Measurement2/LConn1
  Current Measurement2/RConn1 -- Mtc/RConn1

== system Test_FourMotor_PID_Ave/Detailed/Synchronous Motor & Drive4/Subsystem ==
  In : Inport
  "+ -> -1" : Gain  Gain=30/pi
  Bus Selector : BusSelector  OutputSignals=Stator current is_a (A),Rotor speed wm (rad/s),Electromagnetic torque Te (N*m)
  Mux1 : Mux  Inputs=2
  Mux2 : Mux  Inputs=3
  Out : Outport  VectorParamsAs1DForOutWhenUnconnected=off
  tag scope: MotorDrive_4=global
  wires:
  In/1 -> Bus Selector/1, Out/1
  "+ -> -1"/1 -> Mux2/2
  [Mot_TReq_SYS_4] -> Mux1/2
  Bus Selector/2 -> "+ -> -1"/1  "<Rotor speed wm (rad/s)>"
  Bus Selector/3 -> Mux1/1  "<Electromagnetic torque Te (N*m)>"
  Mux1/1 -> Mux2/3
  Bus Selector/1 -> Mux2/1  "<Stator current is_a (A)>"
  Mux2/1 -> [MotorDrive_4]

== system Test_FourMotor_PID_Ave/Detailed/Synchronous Motor & Drive4/Subsystem1 ==
  Sig : Inport
  Bus Selector : BusSelector  OutputSignals=Electromagnetic torque Te (N*m)
  Ideal Rotational Motion Sensor : fl_lib/Mechanical/Mechanical Sensors/Ideal Rotational Motion Sensor  reference=foundation.enum.MeasurementReference.difference  acceleration_port=false  velocity_port=true  position_port=true  wrap_angle=simscape.enum.onoff.off  offset=0 rad
  Ideal Torque Source : fl_lib/Mechanical/Mechanical Sources/Ideal Torque Source
  Mechanical Rotational Reference : fl_lib/Mechanical/Rotational Elements/Mechanical Rotational Reference
  Mechanical Rotational Reference1 : fl_lib/Mechanical/Rotational Elements/Mechanical Rotational Reference
  PS-Simulink Converter : nesl_utility/PS-Simulink Converter  PhysicalDomain=network_engine_domain  SubClassName=ps_output  LeftPortType=input  RightPortType=output  PseudoPeriodic=off  Frequencies=[]  VectorFormat=1-D array  Unit=rad/s  AffineConversion=off
  Scope : Scope
      settings: ActiveDisplayYMinimum=-14.945816065975556  ActiveDisplayYMaximum=38.271093163037733  DataLoggingVariableName=ScopeData6
  Simulink-PS Converter : nesl_utility/Simulink-PS Converter  PhysicalDomain=network_engine_domain  SubClassName=ps_input  LeftPortType=input  RightPortType=output  PseudoPeriodic=off  Frequencies=[]  NoiseDistribution=none  NoiseParameters=[]  Unit=1  AffineConversion=off  FilteringAndDerivatives=zero  SimscapeFilterOrder=1  InputFilterTimeConstant=0.005  UdotUserProvided=0
  Sh : PMIOPort  Side=Right
  Spd : Outport  VectorParamsAs1DForOutWhenUnconnected=off
  wires:
  PS-Simulink Converter/1 -> Spd/1
  Sig/1 -> Bus Selector/1
  Bus Selector/1 -> Scope/1, Simulink-PS Converter/1  "<Electromagnetic torque Te (N*m)>"
  connections:
  Simulink-PS Converter/RConn1 -- Ideal Torque Source/RConn1
  PS-Simulink Converter/LConn1 -- Ideal Rotational Motion Sensor/RConn2
  Ideal Rotational Motion Sensor/LConn1 -- Sh/RConn1 -- Ideal Torque Source/LConn1
  Mechanical Rotational Reference1/LConn1 -- Ideal Torque Source/RConn2
  Mechanical Rotational Reference/LConn1 -- Ideal Rotational Motion Sensor/RConn1

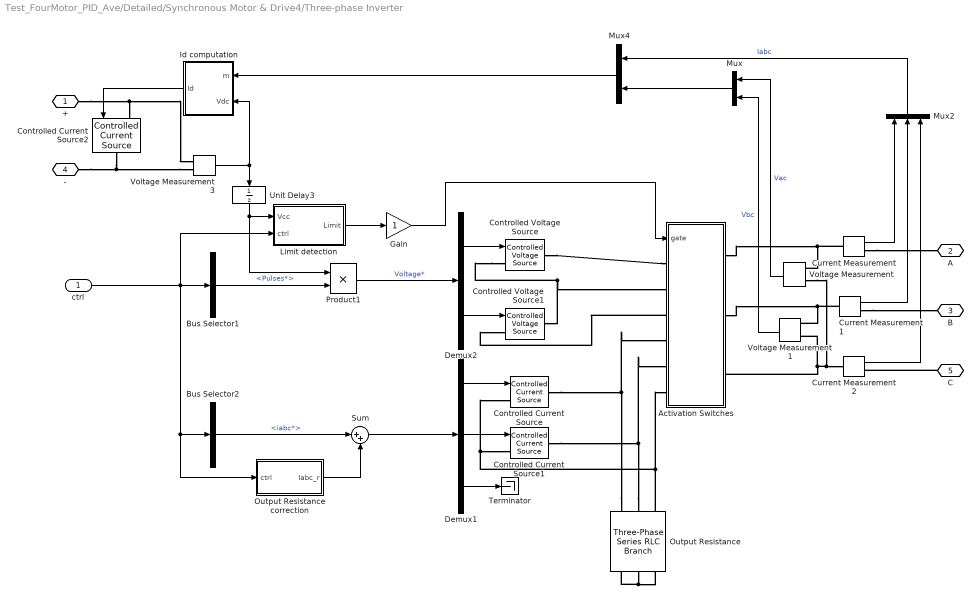
== system Test_FourMotor_PID_Ave/Detailed/Synchronous Motor & Drive4/Three-phase Inverter ==
  ctrl : Inport
  Activation Switches : Subsystem
  Bus Selector1 : BusSelector  OutputSignals=Signals*.Pulses*
  Bus Selector2 : BusSelector  OutputSignals=Signals*.iabc*
  Controlled Current Source : spsControlledCurrentSourceLib/Controlled Current Source  Initialize=on  Source_Type=AC  Amplitude=0  Phase=0  Frequency=0  Measurements=None
  Controlled Current Source1 : spsControlledCurrentSourceLib/Controlled Current Source  Initialize=on  Source_Type=AC  Amplitude=0  Phase=0  Frequency=0  Measurements=None
  Controlled Current Source2 : spsControlledCurrentSourceLib/Controlled Current Source  Initialize=on  Source_Type=AC  Amplitude=0  Phase=0  Frequency=0  Measurements=None
  Controlled Voltage Source : spsControlledVoltageSourceLib/Controlled Voltage Source  Initialize=on  Source_Type=AC  Amplitude=0  Phase=0  Frequency=0  Measurements=None
  Controlled Voltage Source1 : spsControlledVoltageSourceLib/Controlled Voltage Source  Initialize=on  Source_Type=AC  Amplitude=0  Phase=0  Frequency=0  Measurements=None
  Current Measurement : spsCurrentMeasurementLib/Current Measurement  PhasorSimulation=off  OutputType=Complex  PSBequivalent=0
  Current Measurement1 : spsCurrentMeasurementLib/Current Measurement  PhasorSimulation=off  OutputType=Complex  PSBequivalent=0
  Current Measurement2 : spsCurrentMeasurementLib/Current Measurement  PhasorSimulation=off  OutputType=Complex  PSBequivalent=0
  Demux1 : Demux  Outputs=3
      settings: DisplayOption=none
  Demux2 : Demux  Outputs=2
      settings: DisplayOption=none
  Gain : Gain
  Id computation : Subsystem
  Limit detection : Subsystem
  Mux : Mux  Inputs=2
  Mux2 : Mux  Inputs=3
  Mux4 : Mux  Inputs=2
  Output Resistance : spsThreePhaseSeriesRLCBranchLib/Three-Phase Series RLC Branch  LConnTagsString=A|B|C  RConnTagsString=A|B|C  BranchType=R  Resistance=100*Resistance  Inductance=1e-3  Capacitance=1e-6  Measurements=Branch voltages and currents
  Output Resistance correction : Subsystem
  Product1 : Product  RndMeth=Zero
  Sum : Sum  Inputs=|++
  Terminator : Terminator
  Unit Delay3 : UnitDelay  SampleTime=Ts  HasFrameUpgradeWarning=on
  Voltage Measurement : spsVoltageMeasurementLib/Voltage Measurement  PhasorSimulation=off  OutputType=Complex  PSBequivalent=0
  Voltage Measurement1 : spsVoltageMeasurementLib/Voltage Measurement  PhasorSimulation=off  OutputType=Complex  PSBequivalent=0
  Voltage Measurement3 : spsVoltageMeasurementLib/Voltage Measurement  PhasorSimulation=off  OutputType=Complex  PSBequivalent=0
  + : PMIOPort  Side=Right
  A : PMIOPort  Port=2  Side=Left
  B : PMIOPort  Port=3  Side=Left
  - : PMIOPort  Port=4  Side=Right
  C : PMIOPort  Port=5  Side=Left
  wires:
  Current Measurement/1 -> Mux2/1
  Current Measurement1/1 -> Mux2/2
  Voltage Measurement/1 -> Mux/1  "Vac"
  Voltage Measurement1/1 -> Mux/2  "Vbc"
  Mux/1 -> Mux4/2
  Current Measurement2/1 -> Mux2/3
  Mux4/1 -> Id computation/1(m)
  Mux2/1 -> Mux4/1  "Iabc"
  Voltage Measurement3/1 -> Unit Delay3/1, Id computation/2(Vdc)
  Bus Selector1/1 -> Product1/2  "<Pulses*>"
  Demux1/1 -> Controlled Current Source/1
  Demux1/2 -> Controlled Current Source1/1
  Demux1/3 -> Terminator/1
  Demux2/2 -> Controlled Voltage Source1/1
  Demux2/1 -> Controlled Voltage Source/1
  Bus Selector2/1 -> Sum/1  "<iabc*>"
  Limit detection/1(Limit) -> Gain/1
  Sum/1 -> Demux1/1
  Unit Delay3/1 -> Product1/1, Limit detection/1(Vcc)
  ctrl/1 -> Bus Selector1/1, Limit detection/2(ctrl), Bus Selector2/1, Output Resistance correction/1(ctrl)
  Product1/1 -> Demux2/1  "Voltage*"
  Gain/1 -> Activation Switches/1(gate)
  Id computation/1(Id) -> Controlled Current Source2/1
  Output Resistance correction/1("Iabc_r ") -> Sum/2
  connections:
  Voltage Measurement3/LConn1 -- Controlled Current Source2/LConn1 -- +/RConn1
  Voltage Measurement3/LConn2 -- Controlled Current Source2/RConn1 -- -/RConn1
  Activation Switches/LConn6 -- Controlled Current Source/LConn1 -- Controlled Current Source1/LConn1 -- Output Resistance/LConn3
  Output Resistance/RConn1 -- Output Resistance/RConn3 -- Output Resistance/RConn2
  Voltage Measurement/LConn1 -- Activation Switches/RConn1 -- Current Measurement/LConn1
  Output Resistance/LConn1 -- Activation Switches/LConn4 -- Controlled Current Source/RConn1
  Output Resistance/LConn2 -- Activation Switches/LConn5 -- Controlled Current Source1/RConn1
  Voltage Measurement/LConn2 -- Activation Switches/RConn3 -- Voltage Measurement1/LConn2 -- Current Measurement2/LConn1
  Controlled Voltage Source/LConn1 -- Activation Switches/LConn2 -- Controlled Voltage Source1/RConn1
  Voltage Measurement1/LConn1 -- Activation Switches/RConn2 -- Current Measurement1/LConn1
  Current Measurement/RConn1 -- A/RConn1
  Current Measurement1/RConn1 -- B/RConn1
  C/RConn1 -- Current Measurement2/RConn1
  Controlled Voltage Source/RConn1 -- Activation Switches/LConn1
  Activation Switches/LConn3 -- Controlled Voltage Source1/LConn1

== system Test_FourMotor_PID_Ave/Detailed/Synchronous Motor & Drive4/Torque limitation ==
  N rad/s : Inport
  Torque : Inport  Port=2
  Abs1 : Abs
  Gain : Gain  Gain=-1
  Saturation Dynamic : simulink/Discontinuities/Saturation Dynamic  OutMin=[]  OutMax=[]  OutDataTypeStr=Inherit: Same as second input  OutDataType=sfix(16)  OutScaling=2^-10  DoSatur=off
  Torque vs speed profile : Lookup  InputValues=HEV_Param.Motor.TorqSpdLUT.SpeedRPM*pi/30  Table=HEV_Param.Motor.TorqSpdLUT.TorqueNm  LookUpMeth=Interpolation-Use End Values  SaturateOnIntegerOverflow=off
  torque : Outport  VectorParamsAs1DForOutWhenUnconnected=off
  wires:
  Gain/1 -> Saturation Dynamic/3
  Torque/1 -> Saturation Dynamic/2
  Saturation Dynamic/1 -> torque/1
  Torque vs speed profile/1 -> Gain/1, Saturation Dynamic/1
  Abs1/1 -> Torque vs speed profile/1
  N rad/s/1 -> Abs1/1

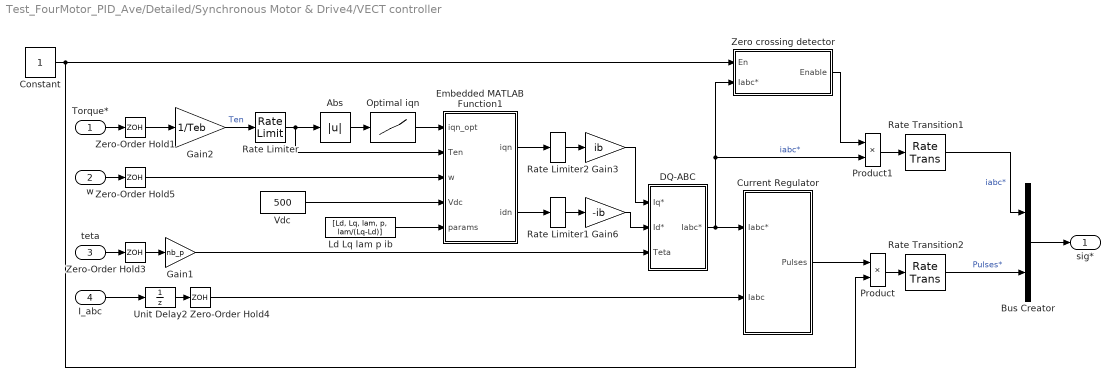
== system Test_FourMotor_PID_Ave/Detailed/Synchronous Motor & Drive4/VECT controller ==
  Torque* : Inport
  w : Inport  Port=2
  teta : Inport  Port=3
  I_abc : Inport  Port=4
  Abs : Abs  SaturateOnIntegerOverflow=off
  Bus Creator : BusCreator  Inputs=2
  Constant : Constant
  Current Regulator : Subsystem
  DQ-ABC : Subsystem
  Embedded MATLAB Function1 : MATLAB Function  TreatAsAtomicUnit=on  SystemSampleTime=Ts_vect
  Gain1 : Gain  Gain=nb_p  SaturateOnIntegerOverflow=on  OutDataTypeStr=Inherit: Same as input  ParamDataTypeStr=Inherit: Same as input
  Gain2 : Gain  Gain=1/Teb  SaturateOnIntegerOverflow=on  OutDataTypeStr=Inherit: Same as input  ParamDataTypeStr=Inherit: Same as input
  Gain3 : Gain  Gain=ib  SaturateOnIntegerOverflow=on  OutDataTypeStr=Inherit: Same as input  ParamDataTypeStr=Inherit: Same as input
  Gain6 : Gain  Gain=-ib  SaturateOnIntegerOverflow=on  OutDataTypeStr=Inherit: Same as input  ParamDataTypeStr=Inherit: Same as input
  Ld Lq lam p ib : Constant  Value=[Ld, Lq, lam, p, lam/(Lq-Ld)]
  Optimal iqn : Lookup  InputValues=ten  Table=iqn  SaturateOnIntegerOverflow=off
  Product : Product  RndMeth=Zero
  Product1 : Product  RndMeth=Zero
  Rate Limiter : RateLimiter  RisingSlewLimit=10  FallingSlewLimit=-10  LinearizeAsGain=off
  Rate Limiter1 : RateLimiter  RisingSlewLimit=100  FallingSlewLimit=-100  SampleTimeMode=inherited
  Rate Limiter2 : RateLimiter  RisingSlewLimit=100  FallingSlewLimit=-100  SampleTimeMode=inherited
  Rate Transition1 : RateTransition
  Rate Transition2 : RateTransition
  Unit Delay2 : UnitDelay  SampleTime=-1  HasFrameUpgradeWarning=on
  Vdc : Constant  Value=500
  Zero crossing detector : Subsystem
  Zero-Order Hold{1,3..5} (4 alike) : ZeroOrderHold  SampleTime=Ts_vect
  sig* : Outport  VectorParamsAs1DForOutWhenUnconnected=off
  wires:
  Unit Delay2/1 -> Zero-Order Hold4/1
  Zero-Order Hold4/1 -> Current Regulator/2(Iabc)
  teta/1 -> Zero-Order Hold3/1
  Zero-Order Hold3/1 -> Gain1/1
  Gain1/1 -> DQ-ABC/3(Teta)
  DQ-ABC/1(Iabc*) -> Current Regulator/1(Iabc*), Zero crossing detector/2(Iabc*), Product1/2  "iabc*"
  I_abc/1 -> Unit Delay2/1
  Torque*/1 -> Zero-Order Hold1/1
  Gain3/1 -> DQ-ABC/1("Iq* ")
  Gain6/1 -> DQ-ABC/2("Id* ")
  Zero-Order Hold1/1 -> Gain2/1
  w/1 -> Zero-Order Hold5/1
  Embedded MATLAB Function1/2(idn) -> Rate Limiter1/1
  Gain2/1 -> Rate Limiter/1  "Ten"
  Zero-Order Hold5/1 -> Embedded MATLAB Function1/3(w)
  Ld Lq lam p ib/1 -> Embedded MATLAB Function1/5(params)
  Embedded MATLAB Function1/1(iqn) -> Rate Limiter2/1
  Optimal iqn/1 -> Embedded MATLAB Function1/1(iqn_opt)
  Abs/1 -> Optimal iqn/1
  Vdc/1 -> Embedded MATLAB Function1/4(Vdc)
  Bus Creator/1 -> sig*/1
  Rate Transition2/1 -> Bus Creator/2  "Pulses*"
  Rate Transition1/1 -> Bus Creator/1  "iabc*"
  Current Regulator/1(Pulses) -> Product/1
  Product/1 -> Rate Transition2/1
  Product1/1 -> Rate Transition1/1
  Zero crossing detector/1(Enable) -> Product1/1
  Constant/1 -> Zero crossing detector/1(En), Product/2
  Rate Limiter2/1 -> Gain3/1
  Rate Limiter1/1 -> Gain6/1
  Rate Limiter/1 -> Abs/1, Embedded MATLAB Function1/2(Ten)

== system Test_FourMotor_PID_Ave/Detailed/DC//DC Converter/PWM/Sawtooth generator ==
  1\ib3 : Gain  Gain=2  SaturateOnIntegerOverflow=on  OutDataTypeStr=Inherit: Same as input  ParamDataTypeStr=Inherit: Same as input
  Constant1 : Constant  Value=20000
  Constant2 : Constant  Value=2
  Constant3 : Constant
  Discrete-Time Integrator : DiscreteIntegrator  IntegratorMethod=Integration: Trapezoidal  ExternalReset=rising  SampleTime=Ts  UpperSaturationLimit=1.5  LowerSaturationLimit=-1.5  ICPrevOutput=DiscIntNeverNeededParam  ICPrevScaledInput=DiscIntNeverNeededParam
  Relational Operator1 : RelationalOperator  InputSameDT=off
  Sum1 : Sum  Inputs=+-  InputSameDT=on  SaturateOnIntegerOverflow=on  OutDataTypeStr=Inherit: Same as first input
  Unit Delay : UnitDelay  SampleTime=Ts  HasFrameUpgradeWarning=on
  Out : Outport  VectorParamsAs1DForOutWhenUnconnected=off
  wires:
  Constant1/1 -> 1\ib3/1
  Discrete-Time Integrator/1 -> Relational Operator1/1, Sum1/1
  Constant2/1 -> Relational Operator1/2
  Relational Operator1/1 -> Unit Delay/1
  Unit Delay/1 -> Discrete-Time Integrator/2
  Sum1/1 -> Out/1
  Constant3/1 -> Sum1/2
  1\ib3/1 -> Discrete-Time Integrator/1

== system Test_FourMotor_PID_Ave/Detailed/DC//DC Converter/PWM/Thermal Model ==
  IBus : Inport
  1/Mc : Gain  Gain=1/(HEV_Param.DCDCConv.Thermal_Mass*HEV_Param.DCDCConv.Specific_Heat)  SaturateOnIntegerOverflow=on  OutDataTypeStr=Inherit: Same as input  ParamDataTypeStr=Inherit: Same as input
  Air_Temp : Constant  Value=HEV_Param.DCDCConv.Air_Temperature-273
  Heat Losses : Gain  Gain=HEV_Param.DCDCConv.Convection.Area/HEV_Param.DCDCConv.Convection.HT_Coefficient  SaturateOnIntegerOverflow=on  OutDataTypeStr=Inherit: Same as input  ParamDataTypeStr=Inherit: Same as input
  Integrator : Integrator  InitialCondition=HEV_Param.DCDCConv.Initial_Temperature
  Subsystem : Subsystem
  Sum1 : Sum  Inputs=|+-  InputSameDT=on  SaturateOnIntegerOverflow=on  OutDataTypeStr=Inherit: Same as first input
  Sum2 : Sum  Inputs=|+-  InputSameDT=on  SaturateOnIntegerOverflow=on  OutDataTypeStr=Inherit: Same as first input
  tag scope: DCDC_SYS=global
  wires:
  Sum1/1 -> 1/Mc/1
  Sum2/1 -> Heat Losses/1
  Heat Losses/1 -> Sum1/2
  1/Mc/1 -> Integrator/1
  Integrator/1 -> [DCDC_SYS], Sum2/1  "DCDC_Temp"
  IBus/1 -> Subsystem/1(IBus)
  Subsystem/1(Heat Flow) -> Sum1/1  "Heat In"
  Air_Temp/1 -> Sum2/2

== system Test_FourMotor_PID_Ave/Detailed/Synchronous Motor & Drive1/Three-phase Inverter/Activation Switches ==
  gate : Inport
  Ideal Switch1 : spsIdealSwitchLib/Ideal Switch  Ron=2*Ron  Lon=0  IC=1  Rs=1e6  Cs=inf  Measurements=off
  Ideal Switch2 : spsIdealSwitchLib/Ideal Switch  Ron=2*Ron  Lon=0  IC=1  Rs=1e6  Cs=inf  Measurements=off
  Ideal Switch3 : spsIdealSwitchLib/Ideal Switch  Ron=2*Ron  Lon=0  IC=1  Rs=1e6  Cs=inf  Measurements=off
  Ideal Switch4 : spsIdealSwitchLib/Ideal Switch  Ron=2*Ron  Lon=0  IC=0  Rs=1e6  Cs=inf  Measurements=off
  Ideal Switch5 : spsIdealSwitchLib/Ideal Switch  Ron=2*Ron  Lon=0  IC=0  Rs=1e6  Cs=inf  Measurements=off
  Ideal Switch6 : spsIdealSwitchLib/Ideal Switch  Ron=2*Ron  Lon=0  IC=0  Rs=1e6  Cs=inf  Measurements=off
  Logical Operator : Logic  Operator=NOT  AllPortsSameDT=off  OutDataTypeStr=boolean
  A1 : PMIOPort  Side=Left
  a : PMIOPort  Port=2  Side=Right
  B1 : PMIOPort  Port=3  Side=Left
  b : PMIOPort  Port=4  Side=Right
  C1 : PMIOPort  Port=5  Side=Left
  c : PMIOPort  Port=6  Side=Right
  A2 : PMIOPort  Port=7  Side=Left
  B2 : PMIOPort  Port=8  Side=Left
  C2 : PMIOPort  Port=9  Side=Left
  wires:
  gate/1 -> Ideal Switch1/1, Ideal Switch2/1, Ideal Switch3/1, Logical Operator/1
  Logical Operator/1 -> Ideal Switch4/1, Ideal Switch5/1, Ideal Switch6/1
  connections:
  A1/RConn1 -- Ideal Switch1/LConn1
  Ideal Switch1/RConn1 -- a/RConn1 -- Ideal Switch4/RConn1
  B1/RConn1 -- Ideal Switch2/LConn1
  Ideal Switch2/RConn1 -- Ideal Switch5/RConn1 -- b/RConn1
  C1/RConn1 -- Ideal Switch3/LConn1
  Ideal Switch3/RConn1 -- Ideal Switch6/RConn1 -- c/RConn1
  A2/RConn1 -- Ideal Switch4/LConn1
  B2/RConn1 -- Ideal Switch5/LConn1
  C2/RConn1 -- Ideal Switch6/LConn1
